simulink model "ControlSystems16"  (R2020b)
settings: Solver=VariableStepAuto  StartTime=0.0  StopTime=155  FixedStep=0.001  MinStep=1e-5
undefined symbols (not defined in the file): DiscIntNeverNeededParam, magnitude
libraries: pid_lib x3, simulink x3
settings Model: Creator=markb  LastModifiedBy=orangejuzi
settings SolverCC: ShapePreserveControl=EnableAll  AlgebraicLoopSolver=LineSearch  MinimalZcImpactIntegration=on
settings DebuggingCC: ReadBeforeWriteMsg=DisableAll  WriteAfterWriteMsg=DisableAll  WriteAfterReadMsg=DisableAll  MaxConsecutiveZCsMsg=warning  MultiTaskDSMMsg=none  ModelReferenceExtraNoncontSigs=warning
settings ModelReferenceCC: UpdateModelReferenceTargets=IfOutOfDate
settings SFSimCC: SFSimEcho=off

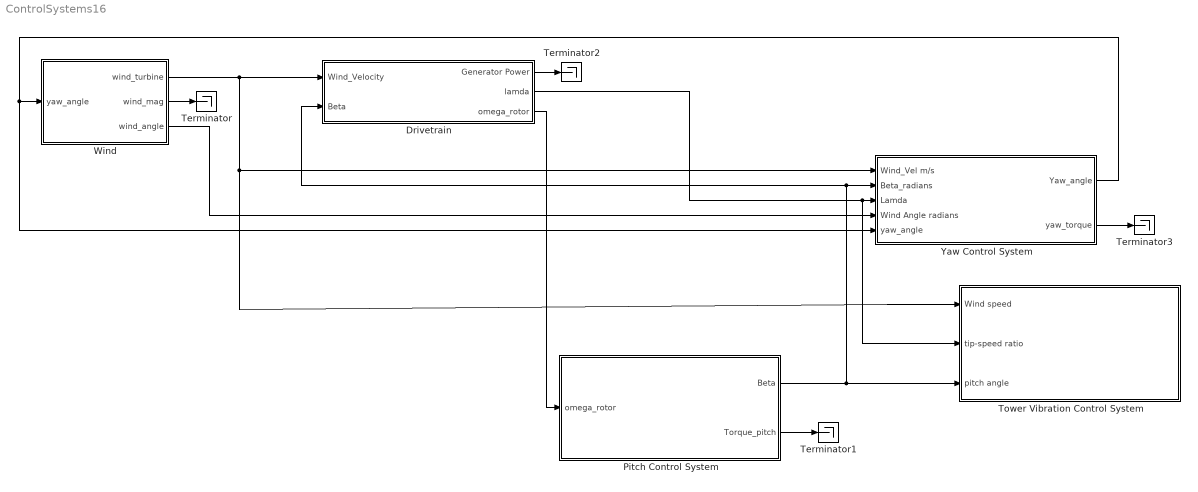
== system ControlSystems16 ==
  Drivetrain : Subsystem
  Pitch Control System : Subsystem
  Terminator{,1..3} (4 alike) : Terminator
  Tower Vibration Control System : Subsystem
  Wind : Subsystem
  Yaw Control System : Subsystem
  wires:
  Yaw Control System/1(Yaw_angle) -> Yaw Control System/5(yaw_angle), Wind/1(yaw_angle)
  Wind/2(wind_mag) -> Terminator/1
  Pitch Control System/1(Beta) -> Drivetrain/2(Beta), Yaw Control System/2(Beta_radians), Tower Vibration Control System/3("pitch angle ")
  Drivetrain/1(Generator Power) -> Terminator2/1
  Wind/3(wind_angle) -> Yaw Control System/4(Wind Angle radians)
  Wind/1(wind_turbine) -> Drivetrain/1(Wind_Velocity), Tower Vibration Control System/1(Wind speed), Yaw Control System/1(Wind_Vel m/s)
  Pitch Control System/2(Torque_pitch) -> Terminator1/1
  Yaw Control System/2(yaw_torque) -> Terminator3/1
  Drivetrain/2(lamda) -> Tower Vibration Control System/2(tip-speed ratio), Yaw Control System/3(Lamda)
  Drivetrain/3(omega_rotor) -> Pitch Control System/1(omega_rotor)

== system ControlSystems16/Drivetrain ==
  Wind_Velocity : Inport
  Beta : Inport  Port=2
  Aerodynamic Block : Subsystem
  Electricl Block : Subsystem
  Mechanical Bock : Subsystem
  Generator Power : Outport
  lamda : Outport  Port=2
  omega_rotor : Outport  Port=3
  wires:
  Mechanical Bock/2(omega_Gen) -> Electricl Block/1(HSS_Speed)
  Electricl Block/2(Generator Torque) -> Mechanical Bock/2(Gen_Torque)
  Mechanical Bock/1(omega_rotor) -> omega_rotor/1, Aerodynamic Block/1(Rotor_Angular_Velocity)
  Wind_Velocity/1 -> Aerodynamic Block/2(Wind_Velocity)
  Beta/1 -> Aerodynamic Block/3(Beta)
  Aerodynamic Block/2(lamda) -> lamda/1
  Aerodynamic Block/1(Rotor_Torque) -> Mechanical Bock/1(Rotor_Torque)
  Electricl Block/1(Generator Power) -> Generator Power/1

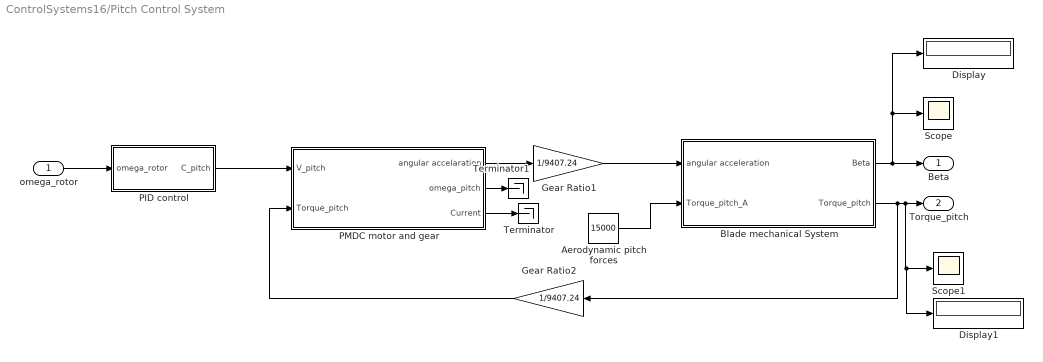
== system ControlSystems16/Pitch Control System ==
  omega_rotor : Inport
  Aerodynamic pitch forces : Constant  Value=15000
  Blade mechanical System : Subsystem
  Display : Display
  Display1 : Display
  Gear Ratio1 : Gain  Gain=1/9407.24
  Gear Ratio2 : Gain  Gain=1/9407.24
  PID control : Subsystem
  PMDC motor and gear : Subsystem
  Scope : Scope
  Scope1 : Scope
  Terminator : Terminator
  Terminator1 : Terminator
  Beta : Outport
  Torque_pitch : Outport  Port=2
  wires:
  omega_rotor/1 -> PID control/1(omega_rotor)
  Aerodynamic pitch forces/1 -> Blade mechanical System/2(Torque_pitch_A)
  Blade mechanical System/2(Torque_pitch) -> Display1/1, Scope1/1, Torque_pitch/1, Gear Ratio2/1
  PID control/1(C_pitch) -> PMDC motor and gear/1(V_pitch)
  Blade mechanical System/1(Beta) -> Display/1, Scope/1, Beta/1
  Gear Ratio1/1 -> Blade mechanical System/1(angular acceleration)
  Gear Ratio2/1 -> PMDC motor and gear/2(Torque_pitch)
  PMDC motor and gear/1(angular accelaration) -> Gear Ratio1/1
  PMDC motor and gear/3(Current) -> Terminator/1
  PMDC motor and gear/2(omega_pitch) -> Terminator1/1

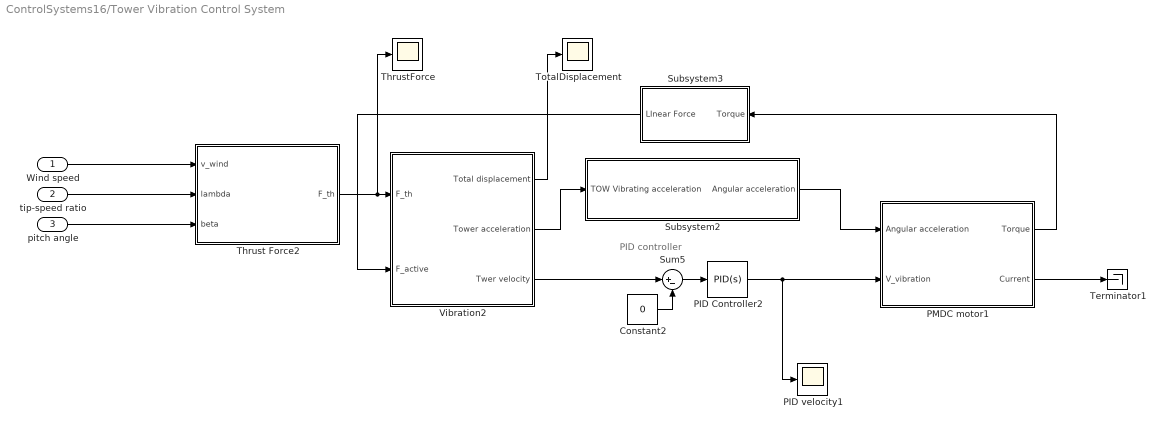
== system ControlSystems16/Tower Vibration Control System ==
  note: PID controller
  Wind speed : Inport
  tip-speed ratio : Inport  Port=2
  "pitch angle " : Inport  Port=3
  Constant2 : Constant  Value=0
  PID Controller2 : pid_lib/PID Controller  Controller=PID  Form=Parallel  TimeDomain=Continuous-time  UseExternalTs=off  SampleTime=-1  IntegratorMethod=Forward Euler  FilterMethod=Forward Euler  ControllerParametersSource=internal  P=-2000  I=-1  D=-1  UseFilter=on  N=597.035100888721  TunerSelectOption=Transfer Function Based (PID Tuner App)  InitialConditionSource=internal  InitialConditionForIntegrator=0  InitialConditionForFilter=0  DifferentiatorICPrevScaledInput=0  ExternalReset=none  TrackingMode=off  Kt=1  LimitOutput=off  SatLimitsSource=internal  UpperSaturationLimit=inf  LowerSaturationLimit=-inf  LinearizeAsGain=on  AntiWindupMode=none  Kb=1  POutMin=[]  POutMax=[]  IOutMin=[]  IOutMax=[]  DOutMin=[]  DOutMax=[]  NOutMin=[]  NOutMax=[]  SumOutMin=[]  SumOutMax=[]  SaturationOutMin=[]  SaturationOutMax=[]  PParamMin=[]  PParamMax=[]  IParamMin=[]  IParamMax=[]  DParamMin=[]  DParamMax=[]  NParamMin=[]  NParamMax=[]  KbParamMin=[]  KbParamMax=[]  KtParamMin=[]  KtParamMax=[]  KbOutMin=[]  KbOutMax=[]  KtOutMin=[]  KtOutMax=[]  IntegratorOutMin=[]  IntegratorOutMax=[]  FilterOutMin=[]  FilterOutMax=[]  SumI1OutMin=[]  SumI1OutMax=[]  SumI2OutMin=[]  SumI2OutMax=[]  SumI3OutMin=[]  SumI3OutMax=[]  SumI4OutMin=[]  SumI4OutMax=[]  SumDOutMin=[]  SumDOutMax=[]  DifferentiatorOutMin=[]  DifferentiatorOutMax=[]  FilterDiffOutCoefMin=[]  FilterDiffOutCoefMax=[]  ReciprocalOutMin=[]  ReciprocalOutMax=[]  SumDenOutMin=[]  SumDenOutMax=[]  SumNumOutMin=[]  SumNumOutMax=[]  DivideOutMin=[]  DivideOutMax=[]  UdiffTsProdOutMin=[]  UdiffTsProdOutMax=[]  NTsProdOutMin=[]  NTsProdOutMax=[]  UintegralTsProdOutMin=[]  UintegralTsProdOutMax=[]  UngainTsProdOutMin=[]  UngainTsProdOutMax=[]  IntegratorContinuousStateAttributes=''  IntegratorStateMustResolveToSignalObject=off  IntegratorRTWStateStorageClass=Auto  FilterContinuousStateAttributes=''  FilterStateMustResolveToSignalObject=off  FilterRTWStateStorageClass=Auto  ParallelPVariant=InternalParameters  IdealPVariant=Disabled  IVariant=InternalParameters  DVariant=InternalParameters  IntegratorVariant=Continuous  SatVariant=Disabled  AWVariant=Passthrough  PCopyVariant=Disabled  TRVariant=Disabled  FdbkBlocksVariant=Forward  IdealPFdbkVariant=Disabled  SatFdbkVariant=Disabled  DerivativeFilterVariant=ContFilter  NVariant=InternalParameters  NCopyVariant=Disabled  FilterICVariant=InternalICsFilter  IntegratorICVariant=InternalICs  ExternalResetVariant=Disabled  TRSumVariant=Passthrough  SumFdbkVariant=Disabled  SumVariant=Sum_PID  TsampFilterVariant=InternalTs  TsampNgainVariant=Passthrough  TsampIntegralVariant=Passthrough  ExternalSaturationOutDataTypeStr=Inherit: Same as second input
  PID velocity1 : Scope
  PMDC motor1 : Subsystem
  Subsystem2 : Subsystem
  Subsystem3 : Subsystem
  Sum5 : Sum  Inputs=|+-
  Terminator1 : Terminator
  Thrust Force2 : Subsystem
  ThrustForce : Scope
  TotalDisplacement : Scope
  Vibration2 : Subsystem
  wires:
  Wind speed/1 -> Thrust Force2/1(v_wind)
  "pitch angle "/1 -> Thrust Force2/3(beta)
  tip-speed ratio/1 -> Thrust Force2/2(lambda)
  PMDC motor1/2(Current) -> Terminator1/1
  Subsystem2/1(Angular acceleration) -> PMDC motor1/1(Angular acceleration)
  Sum5/1 -> PID Controller2/1
  Constant2/1 -> Sum5/2
  Vibration2/3(Twer velocity) -> Sum5/1
  PID Controller2/1 -> PID velocity1/1, PMDC motor1/2(V_vibration)
  PMDC motor1/1(Torque) -> Subsystem3/1(Torque)
  Vibration2/2(Tower acceleration) -> Subsystem2/1(TOW Vibrating acceleration)
  Thrust Force2/1(F_th) -> ThrustForce/1, Vibration2/1(F_th)
  Vibration2/1(Total displacement) -> TotalDisplacement/1
  Subsystem3/1(LInear Force) -> Vibration2/2(F_active)

== system ControlSystems16/Wind ==
  yaw_angle : Inport
  Add : Sum  Inputs=-+
  Product : Product
  Ramp_for_wind_test : simulink/Sources/Ramp  slope=0.1  start=0  InitialOutput=10
  Terminator : Terminator
  Trigonometric Function : Trigonometry  Operator=cos
  Wind_mag : simulink/Sources/Repeating Sequence Interpolated  OutValues=[6 10 15 10 10 15 18 20 22 26 20 22 18 15 13 13 12 10 9 11 17 17 19 19 25 25 26 19 13 10 7 ].'  TimeValues=[0 5 15 20 25 30 35 40 45 50 55 60 65 70 75 80 85 90 95 100 105 110 115 120 125 130 135 140 145 150 155 ].'  LookUpMeth=Interpolation-Use End Values  tsamp=0.01  OutMin=[]  OutMax=[]  OutDataTypeStr=double  OutputDataTypeScalingMode=double  OutDataType=fixdt(0,8)  OutScaling=2^-10
  deg_to_rad : Gain  Gain=pi/180
  omega_w_deg : simulink/Sources/Repeating Sequence Interpolated  OutValues=[ 0 0 0 6 10 12 12 4 8 12 16 16 24 28 24 16 12 4 2 0 0 -2 -4 -4 -10 -14 -18 -20 -12 -8 -4 ].'  TimeValues=[0 5 15 20 25 30 35 40 45 50 55 60 65 70 75 80 85 90 95 100 105 110 115 120 125 130 135 140 145 150 155 ].'  LookUpMeth=Interpolation-Use End Values  tsamp=0.01  OutMin=[]  OutMax=[]  OutDataTypeStr=double  OutputDataTypeScalingMode=double  OutDataType=fixdt(0,8)  OutScaling=2^-10
  wind_turbine : Outport
  wind_mag : Outport  Port=2
  wind_angle : Outport  Port=3
  wires:
  Add/1 -> Trigonometric Function/1
  Trigonometric Function/1 -> Product/1
  deg_to_rad/1 -> wind_angle/1, Add/2
  yaw_angle/1 -> Add/1
  omega_w_deg/1 -> deg_to_rad/1
  Wind_mag/1 -> wind_mag/1, Product/2
  Product/1 -> wind_turbine/1
  Ramp_for_wind_test/1 -> Terminator/1

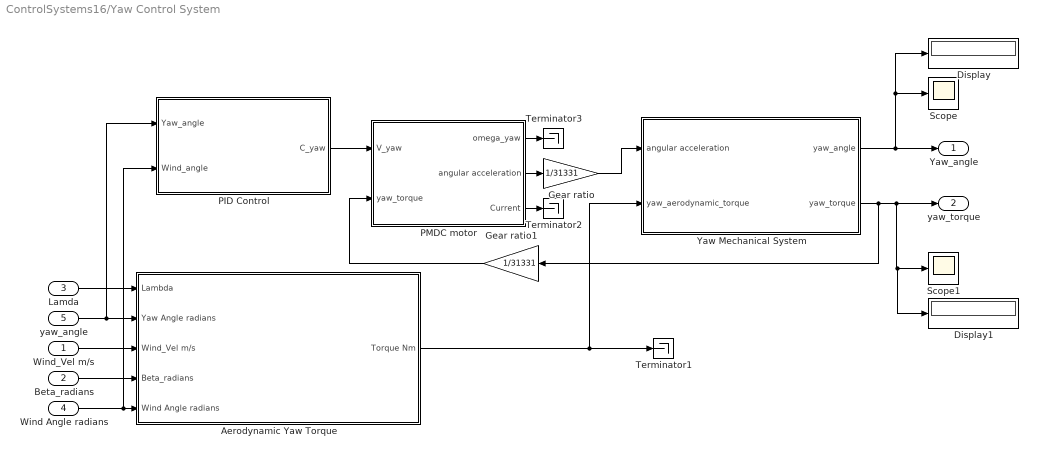
== system ControlSystems16/Yaw Control System ==
  Wind_Vel m/s : Inport
  Beta_radians : Inport  Port=2
  Lamda : Inport  Port=3
  Wind Angle radians : Inport  Port=4
  yaw_angle : Inport  Port=5
  Aerodynamic Yaw Torque : Subsystem
  Display : Display
  Display1 : Display
  Gear ratio : Gain  Gain=1/31331
  Gear ratio1 : Gain  Gain=1/31331
  PID Control : Subsystem
  PMDC motor : Subsystem
  Scope : Scope
  Scope1 : Scope
  Terminator1 : Terminator
  Terminator2 : Terminator
  Terminator3 : Terminator
  Yaw Mechanical System : Subsystem
  Yaw_angle : Outport
  yaw_torque : Outport  Port=2
  wires:
  Wind_Vel m/s/1 -> Aerodynamic Yaw Torque/3(Wind_Vel m/s)
  Wind Angle radians/1 -> PID Control/2(Wind_angle), Aerodynamic Yaw Torque/5(Wind Angle radians)
  Beta_radians/1 -> Aerodynamic Yaw Torque/4(Beta_radians)
  Lamda/1 -> Aerodynamic Yaw Torque/1(Lambda)
  Aerodynamic Yaw Torque/1(Torque Nm) -> Terminator1/1, Yaw Mechanical System/2(yaw_aerodynamic_torque)
  yaw_angle/1 -> Aerodynamic Yaw Torque/2(Yaw Angle radians), PID Control/1(Yaw_angle)
  PID Control/1(C_yaw) -> PMDC motor/1(V_yaw)
  Yaw Mechanical System/2(yaw_torque) -> Display1/1, Scope1/1, yaw_torque/1, Gear ratio1/1
  Yaw Mechanical System/1(yaw_angle) -> Display/1, Scope/1, Yaw_angle/1
  PMDC motor/3(Current) -> Terminator2/1
  PMDC motor/2(angular acceleration) -> Gear ratio/1
  Gear ratio/1 -> Yaw Mechanical System/1(angular acceleration)
  Gear ratio1/1 -> PMDC motor/2(yaw_torque)
  PMDC motor/1(omega_yaw) -> Terminator3/1

== system ControlSystems16/Drivetrain/Aerodynamic Block ==
  Rotor_Angular_Velocity : Inport
  Wind_Velocity : Inport  Port=2
  Beta : Inport  Port=3
  Power Coefficient : Subsystem
  Rotor Torque : Subsystem
  Tip speed Ratio : Subsystem
  Rotor_Torque : Outport
  lamda : Outport  Port=2
  wires:
  Beta/1 -> Power Coefficient/2(Beta)
  Tip speed Ratio/1(Tip_Speed_Ratio) -> lamda/1, Power Coefficient/1(Lamda)
  Power Coefficient/1(C_p) -> Rotor Torque/1(Power_Coefficient)
  Rotor_Angular_Velocity/1 -> Rotor Torque/3(Rotor_Angular_Velocity), Tip speed Ratio/1(Rotor_Angular_Velocity)
  Rotor Torque/1(Rotor_Torque) -> Rotor_Torque/1
  Wind_Velocity/1 -> Rotor Torque/2(Wind_Speed), Tip speed Ratio/2(Wind_Velocity)

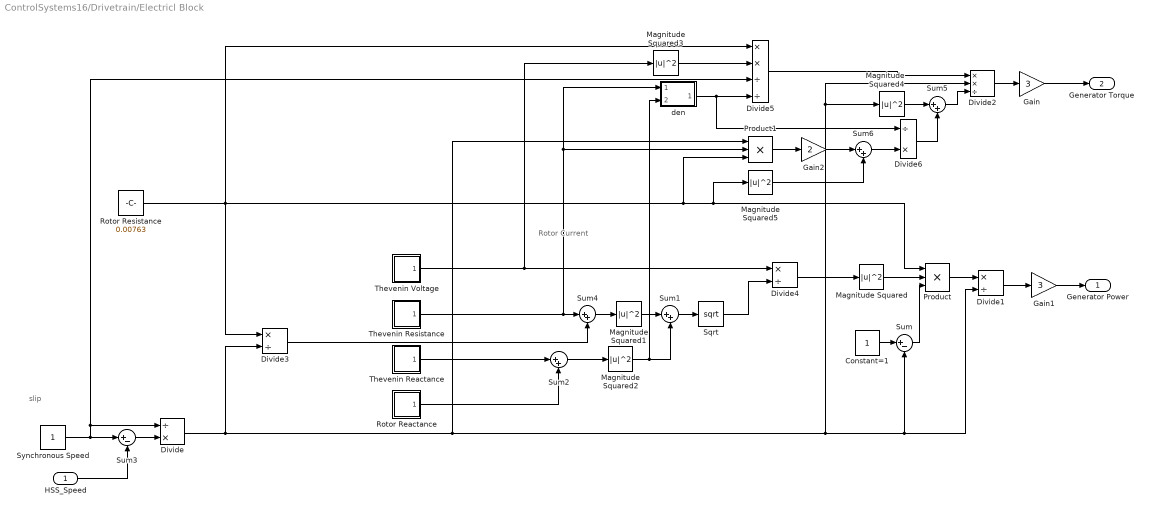
== system ControlSystems16/Drivetrain/Electricl Block ==
  note: slip
  note: Rotor Current
  HSS_Speed : Inport
  Constant=1 : Constant
  Divide : Product  Inputs=/*
  Divide1 : Product  Inputs=*/
  Divide2 : Product  Inputs=**/
  Divide3 : Product  Inputs=*/
  Divide4 : Product  Inputs=*/
  Divide5 : Product  Inputs=**//
  Divide6 : Product  Inputs=/*
  Gain : Gain  Gain=3
  Gain1 : Gain  Gain=3
  Gain2 : Gain  Gain=2
  Magnitude Squared{,1..5} (6 alike) : Math  Operator=magnitude^2  SaturateOnIntegerOverflow=on
  Product : Product  Inputs=3
  Product1 : Product  Inputs=3
  Rotor Reactance : Subsystem
  Rotor Resistance : Constant  Value=0.00763
  Sqrt : Sqrt  SaturateOnIntegerOverflow=on
  Sum : Sum  Inputs=|+-
  Sum{1..2,4..6} (5 alike) : Sum  Inputs=|++
  Sum3 : Sum  Inputs=|+-
  Synchronous Speed : Constant
  Thevenin Reactance : Subsystem
  Thevenin Resistance : Subsystem
  Thevenin Voltage : Subsystem
  den : Subsystem
  Generator Power : Outport
  Generator Torque : Outport  Port=2
  wires:
  Product/1 -> Divide1/1
  Divide1/1 -> Gain1/1
  Gain1/1 -> Generator Power/1
  Sum/1 -> Product/3
  Divide/1 -> Product1/1, Divide1/2, Sum/2, Magnitude Squared4/1, Divide2/2, Divide3/2
  Constant=1/1 -> Sum/1
  Rotor Resistance/1 -> Product1/3, Product/1, Magnitude Squared5/1, Divide3/1, Divide5/1
  Divide4/1 -> Magnitude Squared/1
  Magnitude Squared/1 -> Product/2
  Gain/1 -> Generator Torque/1
  Divide2/1 -> Gain/1
  Thevenin Voltage/1(Out1) -> Magnitude Squared3/1, Divide4/1
  Divide3/1 -> Sum4/2
  Magnitude Squared2/1 -> Sum1/2, den/2(In2)
  Magnitude Squared1/1 -> Sum1/1
  Sqrt/1 -> Divide4/2
  Sum2/1 -> Magnitude Squared2/1
  Thevenin Reactance/1(Out1) -> Sum2/1
  Sum1/1 -> Sqrt/1
  Magnitude Squared3/1 -> Divide5/2
  Synchronous Speed/1 -> Divide5/3, Divide/1, Sum3/1
  HSS_Speed/1 -> Sum3/2
  Sum3/1 -> Divide/2
  Divide5/1 -> Divide2/1
  den/1(Out1) -> Divide6/1, Divide5/4
  Sum4/1 -> Magnitude Squared1/1
  Sum5/1 -> Divide2/3
  Magnitude Squared4/1 -> Sum5/1
  Divide6/1 -> Sum5/2
  Sum6/1 -> Divide6/2
  Gain2/1 -> Sum6/1
  Product1/1 -> Gain2/1
  Magnitude Squared5/1 -> Sum6/2
  Rotor Reactance/1(Out1) -> Sum2/2
  Thevenin Resistance/1(Out1) -> Sum4/1, Product1/2, den/1(In1)

== system ControlSystems16/Drivetrain/Mechanical Bock ==
  Rotor_Torque : Inport
  Gen_Torque : Inport  Port=2
  Discrete-Time Integrator : DiscreteIntegrator  InitialCondition=1.9  SampleTime=-1  ICPrevOutput=DiscIntNeverNeededParam  ICPrevScaledInput=DiscIntNeverNeededParam
  Gain1 : Gain  Gain=1/(2953248-56.442*80^2)
  Gain2 : Gain  Gain=(2953248-56.442*80^2)/(10-1.6*80^2)
  Gear ratio : Gain  Gain=80
  Gear ratio1 : Gain  Gain=80
  Scope : Scope
  Sum : Sum  Inputs=|+--
  omega_rotor : Outport
  omega_Gen : Outport  Port=2
  wires:
  Rotor_Torque/1 -> Sum/1
  Gen_Torque/1 -> Gear ratio/1
  Gear ratio/1 -> Sum/2
  Gain2/1 -> Sum/3
  Gear ratio1/1 -> omega_Gen/1
  Discrete-Time Integrator/1 -> omega_rotor/1, Scope/1, Gear ratio1/1, Gain2/1
  Sum/1 -> Gain1/1
  Gain1/1 -> Discrete-Time Integrator/1

== system ControlSystems16/Pitch Control System/Blade mechanical System ==
  angular acceleration : Inport
  Torque_pitch_A : Inport  Port=2
  Add : Sum  Inputs=++-
  D_pitch : Gain  Gain=100
  Integrator : Integrator
  Integrator1 : Integrator
  Integrator2 : Integrator
  J_pitch : Gain  Gain=22800
  Beta : Outport
  Torque_pitch : Outport  Port=2
  wires:
  Integrator/1 -> Beta/1
  Add/1 -> Torque_pitch/1
  Torque_pitch_A/1 -> Add/3
  D_pitch/1 -> Add/2
  J_pitch/1 -> Add/1
  angular acceleration/1 -> J_pitch/1, Integrator1/1, Integrator2/1
  Integrator1/1 -> D_pitch/1
  Integrator2/1 -> Integrator/1

== system ControlSystems16/Pitch Control System/PID control ==
  omega_rotor : Inport
  Constant : Constant
  PID Controller : pid_lib/PID Controller  Controller=PID  Form=Parallel  TimeDomain=Continuous-time  UseExternalTs=off  SampleTime=-1  IntegratorMethod=Forward Euler  FilterMethod=Forward Euler  ControllerParametersSource=internal  P=1  I=1  D=0  UseFilter=on  N=100  TunerSelectOption=Transfer Function Based (PID Tuner App)  InitialConditionSource=internal  InitialConditionForIntegrator=0  InitialConditionForFilter=0  DifferentiatorICPrevScaledInput=0  ExternalReset=none  TrackingMode=off  Kt=1  LimitOutput=off  SatLimitsSource=internal  UpperSaturationLimit=inf  LowerSaturationLimit=-inf  LinearizeAsGain=on  AntiWindupMode=none  Kb=1  POutMin=[]  POutMax=[]  IOutMin=[]  IOutMax=[]  DOutMin=[]  DOutMax=[]  NOutMin=[]  NOutMax=[]  SumOutMin=[]  SumOutMax=[]  SaturationOutMin=[]  SaturationOutMax=[]  PParamMin=[]  PParamMax=[]  IParamMin=[]  IParamMax=[]  DParamMin=[]  DParamMax=[]  NParamMin=[]  NParamMax=[]  KbParamMin=[]  KbParamMax=[]  KtParamMin=[]  KtParamMax=[]  KbOutMin=[]  KbOutMax=[]  KtOutMin=[]  KtOutMax=[]  IntegratorOutMin=[]  IntegratorOutMax=[]  FilterOutMin=[]  FilterOutMax=[]  SumI1OutMin=[]  SumI1OutMax=[]  SumI2OutMin=[]  SumI2OutMax=[]  SumI3OutMin=[]  SumI3OutMax=[]  SumI4OutMin=[]  SumI4OutMax=[]  SumDOutMin=[]  SumDOutMax=[]  DifferentiatorOutMin=[]  DifferentiatorOutMax=[]  FilterDiffOutCoefMin=[]  FilterDiffOutCoefMax=[]  ReciprocalOutMin=[]  ReciprocalOutMax=[]  SumDenOutMin=[]  SumDenOutMax=[]  SumNumOutMin=[]  SumNumOutMax=[]  DivideOutMin=[]  DivideOutMax=[]  UdiffTsProdOutMin=[]  UdiffTsProdOutMax=[]  NTsProdOutMin=[]  NTsProdOutMax=[]  UintegralTsProdOutMin=[]  UintegralTsProdOutMax=[]  UngainTsProdOutMin=[]  UngainTsProdOutMax=[]  IntegratorContinuousStateAttributes=''  IntegratorStateMustResolveToSignalObject=off  IntegratorRTWStateStorageClass=Auto  FilterContinuousStateAttributes=''  FilterStateMustResolveToSignalObject=off  FilterRTWStateStorageClass=Auto  ParallelPVariant=InternalParameters  IdealPVariant=Disabled  IVariant=InternalParameters  DVariant=InternalParameters  IntegratorVariant=Continuous  SatVariant=Disabled  AWVariant=Passthrough  PCopyVariant=Disabled  TRVariant=Disabled  FdbkBlocksVariant=Forward  IdealPFdbkVariant=Disabled  SatFdbkVariant=Disabled  DerivativeFilterVariant=ContFilter  NVariant=InternalParameters  NCopyVariant=Disabled  FilterICVariant=InternalICsFilter  IntegratorICVariant=InternalICs  ExternalResetVariant=Disabled  TRSumVariant=Passthrough  SumFdbkVariant=Disabled  SumVariant=Sum_PID  TsampFilterVariant=InternalTs  TsampNgainVariant=Passthrough  TsampIntegralVariant=Passthrough  ExternalSaturationOutDataTypeStr=Inherit: Same as second input
  Sum : Sum  Inputs=|+-
  C_pitch : Outport
  wires:
  omega_rotor/1 -> Sum/1
  PID Controller/1 -> C_pitch/1
  Sum/1 -> PID Controller/1
  Constant/1 -> Sum/2

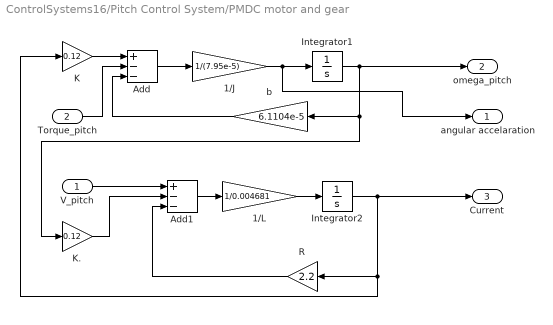
== system ControlSystems16/Pitch Control System/PMDC motor and gear ==
  V_pitch : Inport
  Torque_pitch : Inport  Port=2
  1/J : Gain  Gain=1/(7.95e-5)
  1/L : Gain  Gain=1/0.004681
  Add : Sum  Inputs=+--
  Add1 : Sum  Inputs=+--
  Integrator1 : Integrator
  Integrator2 : Integrator
  K : Gain  Gain=0.12
  K. : Gain  Gain=0.12
  R : Gain  Gain=2.2
  b : Gain  Gain=6.1104e-5
  angular accelaration : Outport
  omega_pitch : Outport  Port=2
  Current : Outport  Port=3
  wires:
  K/1 -> Add/1
  K./1 -> Add1/2
  Add1/1 -> 1/L/1
  Torque_pitch/1 -> Add/2
  Integrator1/1 -> omega_pitch/1, K./1, b/1
  1/L/1 -> Integrator2/1
  1/J/1 -> angular accelaration/1, Integrator1/1
  R/1 -> Add1/3
  Add/1 -> 1/J/1
  Integrator2/1 -> Current/1, R/1, K/1
  V_pitch/1 -> Add1/1
  b/1 -> Add/3

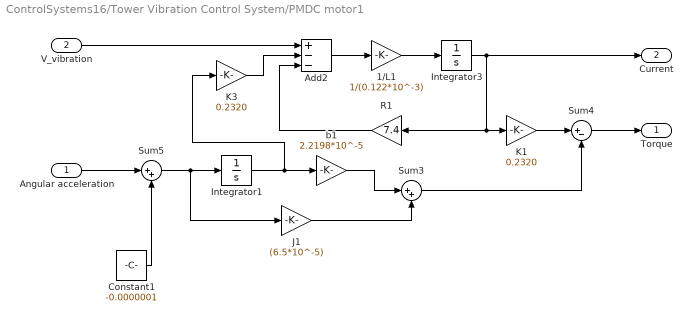
== system ControlSystems16/Tower Vibration Control System/PMDC motor1 ==
  Angular acceleration : Inport
  V_vibration : Inport  Port=2
  1/L1 : Gain  Gain=1/(0.122*10^-3)
  Add2 : Sum  Inputs=+--
  Constant1 : Constant  Value=-0.0000001
  Integrator1 : Integrator
  Integrator3 : Integrator
  J1 : Gain  Gain=(6.5*10^-5)
  K1 : Gain  Gain=0.2320
  K3 : Gain  Gain=0.2320
  R1 : Gain  Gain=7.4
  Sum3 : Sum  Inputs=|++
  Sum4 : Sum  Inputs=|+-
  Sum5 : Sum  Inputs=|++
  b1 : Gain  Gain=2.2198*10^-5
  Torque : Outport
  Current : Outport  Port=2
  wires:
  K3/1 -> Add2/2
  Sum4/1 -> Torque/1
  Add2/1 -> 1/L1/1
  K1/1 -> Sum4/1
  V_vibration/1 -> Add2/1
  Integrator3/1 -> Current/1, R1/1, K1/1
  Constant1/1 -> Sum5/2
  Sum5/1 -> J1/1, Integrator1/1
  Integrator1/1 -> K3/1, b1/1
  1/L1/1 -> Integrator3/1
  b1/1 -> Sum3/1
  Sum3/1 -> Sum4/2
  R1/1 -> Add2/3
  J1/1 -> Sum3/2
  Angular acceleration/1 -> Sum5/1

== system ControlSystems16/Tower Vibration Control System/Subsystem2 ==
  TOW Vibrating acceleration : Inport
  GearRatio : Gain  Gain=1/300
  Angular acceleration : Outport
  wires:
  TOW Vibrating acceleration/1 -> GearRatio/1
  GearRatio/1 -> Angular acceleration/1

== system ControlSystems16/Tower Vibration Control System/Subsystem3 ==
  Torque : Inport
  Raduis : Gain  Gain=4000*0.5
  LInear Force : Outport
  wires:
  Torque/1 -> Raduis/1
  Raduis/1 -> LInear Force/1

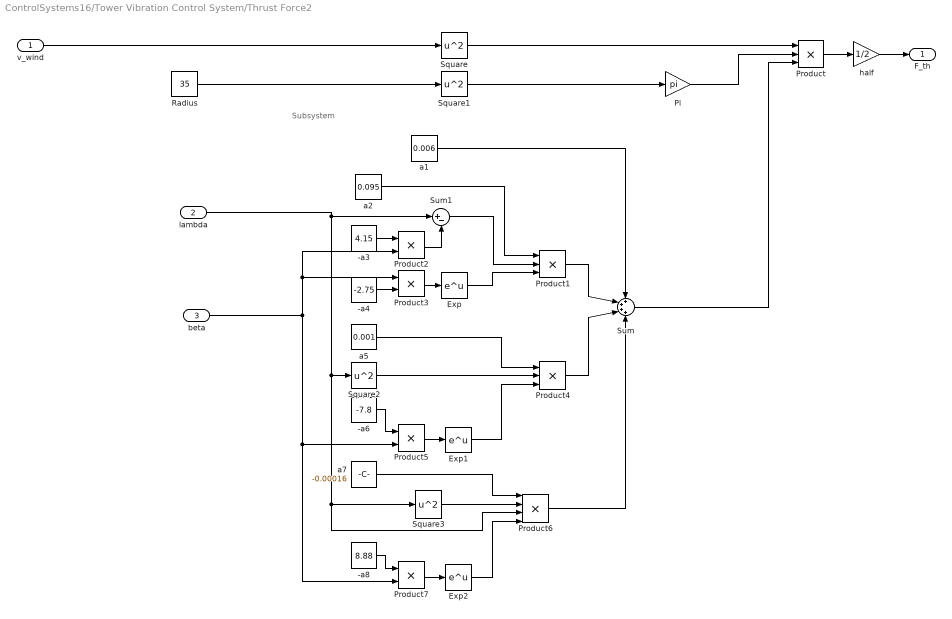
== system ControlSystems16/Tower Vibration Control System/Thrust Force2 ==
  note: Subsystem
  v_wind : Inport
  lambda : Inport  Port=2
  beta : Inport  Port=3
  -a3 : Constant  Value=4.15
  -a4 : Constant  Value=-2.75
  -a6 : Constant  Value=-7.8
  -a8 : Constant  Value=8.88
  Exp : Math  SaturateOnIntegerOverflow=on
  Exp1 : Math  SaturateOnIntegerOverflow=on
  Exp2 : Math  SaturateOnIntegerOverflow=on
  Pi : Gain  Gain=pi
  Product : Product  Inputs=3
  Product1 : Product  Inputs=3
  Product{2..3,5,7} (4 alike) : Product
  Product4 : Product  Inputs=3
  Product6 : Product  Inputs=4
  Radius : Constant  Value=35
  Square{,1..3} (4 alike) : Math  Operator=square  SaturateOnIntegerOverflow=on
  Sum : Sum  Inputs=4
  Sum1 : Sum  Inputs=|+-
  a1 : Constant  Value=0.006
  a2 : Constant  Value=0.095
  a5 : Constant  Value=0.001
  a7 : Constant  Value=-0.00016
  half : Gain  Gain=1/2
  F_th : Outport
  wires:
  v_wind/1 -> Square/1
  half/1 -> F_th/1
  Product/1 -> half/1
  Square/1 -> Product/1
  Radius/1 -> Square1/1
  Square1/1 -> Pi/1
  Pi/1 -> Product/2
  Sum/1 -> Product/3
  Product3/1 -> Exp/1
  Product7/1 -> Exp2/1
  Exp2/1 -> Product6/4
  Exp/1 -> Product1/3
  Product1/1 -> Sum/2
  Product5/1 -> Exp1/1
  lambda/1 -> Square3/1, Product6/3, Square2/1, Sum1/1
  Product2/1 -> Sum1/2
  Product6/1 -> Sum/4
  Exp1/1 -> Product4/3
  Sum1/1 -> Product1/2
  -a6/1 -> Product5/1
  a5/1 -> Product4/1
  Square2/1 -> Product4/2
  a1/1 -> Sum/1
  a2/1 -> Product1/1
  -a8/1 -> Product7/1
  Product4/1 -> Sum/3
  a7/1 -> Product6/1
  -a4/1 -> Product3/2
  -a3/1 -> Product2/1
  beta/1 -> Product5/2, Product7/2, Product3/1, Product2/2
  Square3/1 -> Product6/2

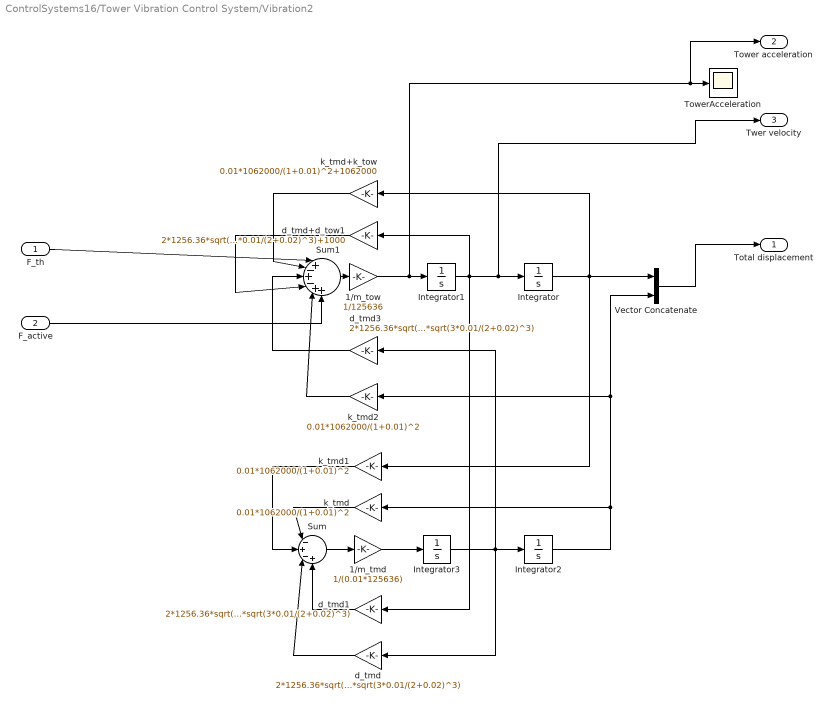
== system ControlSystems16/Tower Vibration Control System/Vibration2 ==
  F_th : Inport
  F_active : Inport  Port=2
  1/m_tmd : Gain  Gain=1/(0.01*125636)
  1/m_tow : Gain  Gain=1/125636
  Integrator : Integrator
  Integrator1 : Integrator  InitialCondition=1.9  UpperSaturationLimit=10  LowerSaturationLimit=-10  AbsoluteTolerance=0.001
  Integrator2 : Integrator
  Integrator3 : Integrator
  Sum : Sum  Inputs=|-+-+
  Sum1 : Sum  Inputs=|+-+-++
  TowerAcceleration : Scope
  Vector Concatenate : Concatenate
  d_tmd : Gain  Gain=2*1256.36*sqrt(1062000/125636)*sqrt(3*0.01/(2+0.02)^3)
  d_tmd+d_tow1 : Gain  Gain=2*1256.36*sqrt(1062000/125636)*sqrt(3*0.01/(2+0.02)^3)+1000
  d_tmd1 : Gain  Gain=2*1256.36*sqrt(1062000/125636)*sqrt(3*0.01/(2+0.02)^3)
  d_tmd3 : Gain  Gain=2*1256.36*sqrt(1062000/125636)*sqrt(3*0.01/(2+0.02)^3)
  k_tmd : Gain  Gain=0.01*1062000/(1+0.01)^2
  k_tmd+k_tow : Gain  Gain=0.01*1062000/(1+0.01)^2+1062000
  k_tmd1 : Gain  Gain=0.01*1062000/(1+0.01)^2
  k_tmd2 : Gain  Gain=0.01*1062000/(1+0.01)^2
  Total displacement : Outport
  Tower acceleration : Outport  Port=2
  Twer velocity : Outport  Port=3
  wires:
  Integrator/1 -> k_tmd+k_tow/1, Vector Concatenate/1, k_tmd1/1
  Integrator3/1 -> d_tmd/1, d_tmd3/1, Integrator2/1
  1/m_tmd/1 -> Integrator3/1
  Sum/1 -> 1/m_tmd/1
  1/m_tow/1 -> Tower acceleration/1, TowerAcceleration/1, Integrator1/1
  Sum1/1 -> 1/m_tow/1
  k_tmd/1 -> Sum/1
  d_tmd/1 -> Sum/3
  d_tmd1/1 -> Sum/4
  k_tmd1/1 -> Sum/2
  k_tmd+k_tow/1 -> Sum1/2
  d_tmd+d_tow1/1 -> Sum1/4
  d_tmd3/1 -> Sum1/3
  Integrator2/1 -> k_tmd/1, k_tmd2/1, Vector Concatenate/2
  k_tmd2/1 -> Sum1/5
  Vector Concatenate/1 -> Total displacement/1
  F_th/1 -> Sum1/1
  F_active/1 -> Sum1/6
  Integrator1/1 -> d_tmd+d_tow1/1, d_tmd1/1, Twer velocity/1, Integrator/1

== system ControlSystems16/Yaw Control System/Aerodynamic Yaw Torque ==
  note: Beta needs to be in radians
  Lambda : Inport
  Yaw Angle radians : Inport  Port=2
  Wind_Vel m/s : Inport  Port=3
  Beta_radians : Inport  Port=4
  Wind Angle radians : Inport  Port=5
  Subtract : Sum  Inputs=+-
  block 1 : Subsystem
  block 2 : Subsystem
  Torque Nm : Outport
  wires:
  block 1/1(C_t) -> block 2/1(Thrust_Coefficient)
  Beta_radians/1 -> block 1/2(beta)
  Wind Angle radians/1 -> Subtract/1
  Yaw Angle radians/1 -> Subtract/2
  Subtract/1 -> block 2/3(Wind Angle difference)
  block 2/1(Yaw_Torque) -> Torque Nm/1
  Lambda/1 -> block 1/1(lambda)
  Wind_Vel m/s/1 -> block 2/2(wind_velocity)

== system ControlSystems16/Yaw Control System/PID Control ==
  Yaw_angle : Inport
  Wind_angle : Inport  Port=2
  Constant : Constant
  PID Controller : pid_lib/PID Controller  Controller=PID  Form=Parallel  TimeDomain=Continuous-time  UseExternalTs=off  SampleTime=-1  IntegratorMethod=Forward Euler  FilterMethod=Forward Euler  ControllerParametersSource=internal  P=3  I=3  D=0  UseFilter=on  N=100  TunerSelectOption=Transfer Function Based (PID Tuner App)  InitialConditionSource=internal  InitialConditionForIntegrator=0  InitialConditionForFilter=0  DifferentiatorICPrevScaledInput=0  ExternalReset=none  TrackingMode=off  Kt=1  LimitOutput=off  SatLimitsSource=internal  UpperSaturationLimit=inf  LowerSaturationLimit=-inf  LinearizeAsGain=on  AntiWindupMode=none  Kb=1  POutMin=[]  POutMax=[]  IOutMin=[]  IOutMax=[]  DOutMin=[]  DOutMax=[]  NOutMin=[]  NOutMax=[]  SumOutMin=[]  SumOutMax=[]  SaturationOutMin=[]  SaturationOutMax=[]  PParamMin=[]  PParamMax=[]  IParamMin=[]  IParamMax=[]  DParamMin=[]  DParamMax=[]  NParamMin=[]  NParamMax=[]  KbParamMin=[]  KbParamMax=[]  KtParamMin=[]  KtParamMax=[]  KbOutMin=[]  KbOutMax=[]  KtOutMin=[]  KtOutMax=[]  IntegratorOutMin=[]  IntegratorOutMax=[]  FilterOutMin=[]  FilterOutMax=[]  SumI1OutMin=[]  SumI1OutMax=[]  SumI2OutMin=[]  SumI2OutMax=[]  SumI3OutMin=[]  SumI3OutMax=[]  SumI4OutMin=[]  SumI4OutMax=[]  SumDOutMin=[]  SumDOutMax=[]  DifferentiatorOutMin=[]  DifferentiatorOutMax=[]  FilterDiffOutCoefMin=[]  FilterDiffOutCoefMax=[]  ReciprocalOutMin=[]  ReciprocalOutMax=[]  SumDenOutMin=[]  SumDenOutMax=[]  SumNumOutMin=[]  SumNumOutMax=[]  DivideOutMin=[]  DivideOutMax=[]  UdiffTsProdOutMin=[]  UdiffTsProdOutMax=[]  NTsProdOutMin=[]  NTsProdOutMax=[]  UintegralTsProdOutMin=[]  UintegralTsProdOutMax=[]  UngainTsProdOutMin=[]  UngainTsProdOutMax=[]  IntegratorContinuousStateAttributes=''  IntegratorStateMustResolveToSignalObject=off  IntegratorRTWStateStorageClass=Auto  FilterContinuousStateAttributes=''  FilterStateMustResolveToSignalObject=off  FilterRTWStateStorageClass=Auto  ParallelPVariant=InternalParameters  IdealPVariant=Disabled  IVariant=InternalParameters  DVariant=InternalParameters  IntegratorVariant=Continuous  SatVariant=Disabled  AWVariant=Passthrough  PCopyVariant=Disabled  TRVariant=Disabled  FdbkBlocksVariant=Forward  IdealPFdbkVariant=Disabled  SatFdbkVariant=Disabled  DerivativeFilterVariant=ContFilter  NVariant=InternalParameters  NCopyVariant=Disabled  FilterICVariant=InternalICsFilter  IntegratorICVariant=InternalICs  ExternalResetVariant=Disabled  TRSumVariant=Passthrough  SumFdbkVariant=Disabled  SumVariant=Sum_PID  TsampFilterVariant=InternalTs  TsampNgainVariant=Passthrough  TsampIntegralVariant=Passthrough  ExternalSaturationOutDataTypeStr=Inherit: Same as second input
  Sum : Sum  Inputs=|-+-
  C_yaw : Outport
  wires:
  Wind_angle/1 -> Sum/2
  Yaw_angle/1 -> Sum/1
  Sum/1 -> PID Controller/1
  Constant/1 -> Sum/3
  PID Controller/1 -> C_yaw/1

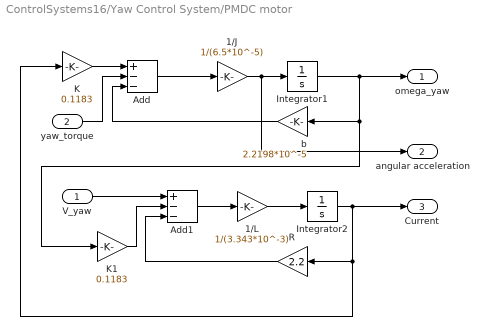
== system ControlSystems16/Yaw Control System/PMDC motor ==
  V_yaw : Inport
  yaw_torque : Inport  Port=2
  1/J : Gain  Gain=1/(6.5*10^-5)
  1/L : Gain  Gain=1/(3.343*10^-3)
  Add : Sum  Inputs=+--
  Add1 : Sum  Inputs=+--
  Integrator1 : Integrator
  Integrator2 : Integrator
  K : Gain  Gain=0.1183
  K1 : Gain  Gain=0.1183
  R : Gain  Gain=2.2
  b : Gain  Gain=2.2198*10^-5
  omega_yaw : Outport
  angular acceleration : Outport  Port=2
  Current : Outport  Port=3
  wires:
  1/J/1 -> angular acceleration/1, Integrator1/1
  Integrator1/1 -> omega_yaw/1, K1/1, b/1
  K1/1 -> Add1/2
  1/L/1 -> Integrator2/1
  yaw_torque/1 -> Add/2
  Add1/1 -> 1/L/1
  K/1 -> Add/1
  Integrator2/1 -> Current/1, R/1, K/1
  b/1 -> Add/3
  Add/1 -> 1/J/1
  V_yaw/1 -> Add1/1
  R/1 -> Add1/3

== system ControlSystems16/Yaw Control System/Yaw Mechanical System ==
  angular acceleration : Inport
  yaw_aerodynamic_torque : Inport  Port=2
  Add : Sum  Inputs=3
  D_yaw : Gain  Gain=200
  Integrator : Integrator
  Integrator1 : Integrator
  Integrator2 : Integrator
  J_yaw : Gain  Gain=45377
  yaw_angle : Outport
  yaw_torque : Outport  Port=2
  wires:
  Integrator/1 -> yaw_angle/1
  Add/1 -> yaw_torque/1
  D_yaw/1 -> Add/2
  yaw_aerodynamic_torque/1 -> Add/3
  J_yaw/1 -> Add/1
  angular acceleration/1 -> Integrator1/1, J_yaw/1, Integrator2/1
  Integrator1/1 -> D_yaw/1
  Integrator2/1 -> Integrator/1

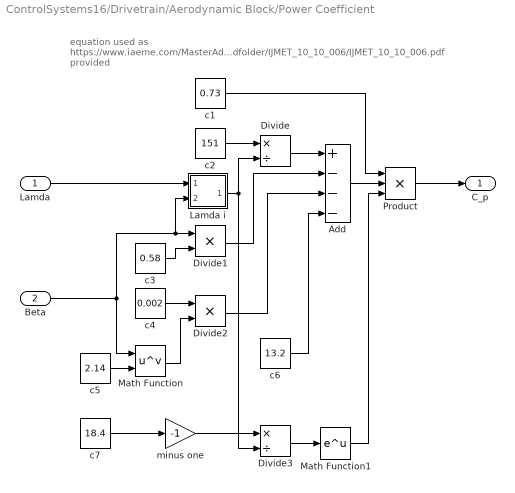
== system ControlSystems16/Drivetrain/Aerodynamic Block/Power Coefficient ==
  note: equation used as
      | https://www.iaeme.com/MasterAdmin/uploadfolder/IJMET_10_10_006/IJMET_10_10_006.pdf provided
  Lamda : Inport
  Beta : Inport  Port=2
  Add : Sum  Inputs=+---
  Divide : Product  Inputs=*/
  Divide1 : Product  Inputs=**
  Divide2 : Product  Inputs=**
  Divide3 : Product  Inputs=*/
  Lamda i : Subsystem
  Math Function : Math  Operator=pow  SaturateOnIntegerOverflow=on
  Math Function1 : Math  SaturateOnIntegerOverflow=on
  Product : Product  Inputs=3
  c1 : Constant  Value=0.73
  c2 : Constant  Value=151
  c3 : Constant  Value=0.58
  c4 : Constant  Value=0.002
  c5 : Constant  Value=2.14
  c6 : Constant  Value=13.2
  c7 : Constant  Value=18.4
  minus one : Gain  Gain=-1
  C_p : Outport
  wires:
  Lamda/1 -> Lamda i/1(In1)
  Beta/1 -> Math Function/1, Divide1/1, Lamda i/2(In2)
  c1/1 -> Product/1
  Product/1 -> C_p/1
  Add/1 -> Product/2
  c2/1 -> Divide/1
  Divide/1 -> Add/1
  Lamda i/1(Out1) -> Divide3/2, Divide/2
  c3/1 -> Divide1/2
  Divide1/1 -> Add/2
  c4/1 -> Divide2/1
  Math Function/1 -> Divide2/2
  c5/1 -> Math Function/2
  Divide2/1 -> Add/3
  c6/1 -> Add/4
  Divide3/1 -> Math Function1/1
  c7/1 -> minus one/1
  minus one/1 -> Divide3/1
  Math Function1/1 -> Product/3

== system ControlSystems16/Drivetrain/Aerodynamic Block/Rotor Torque ==
  note: Power of wind
  Power_Coefficient : Inport
  Wind_Speed : Inport  Port=2
  Rotor_Angular_Velocity : Inport  Port=3
  Divide : Product  Inputs=**/
  Gain : Gain  Gain=0.5*1.225*pi*35^2
  Product : Product
  Square : Math  Operator=square  SaturateOnIntegerOverflow=on
  Rotor_Torque : Outport
  wires:
  Rotor_Angular_Velocity/1 -> Divide/3  "omega_rotor"
  Power_Coefficient/1 -> Divide/1
  Divide/1 -> Rotor_Torque/1
  Wind_Speed/1 -> Square/1, Product/1  "V_wind"
  Gain/1 -> Divide/2
  Product/1 -> Gain/1
  Square/1 -> Product/2

== system ControlSystems16/Drivetrain/Aerodynamic Block/Tip speed Ratio ==
  Rotor_Angular_Velocity : Inport
  Wind_Velocity : Inport  Port=2
  Divide : Product  Inputs=*/
  Radius : Gain  Gain=35
  Tip_Speed_Ratio : Outport
  wires:
  Rotor_Angular_Velocity/1 -> Radius/1  "omega_r"
  Radius/1 -> Divide/1
  Wind_Velocity/1 -> Divide/2  "V_wind"
  Divide/1 -> Tip_Speed_Ratio/1

== system ControlSystems16/Drivetrain/Electricl Block/Rotor Reactance ==
  Gain3 : Gain  Gain=2*pi
  Rotor Inductance : Constant  Value=0.000195
  Out1 : Outport
  wires:
  Gain3/1 -> Out1/1
  Rotor Inductance/1 -> Gain3/1

== system ControlSystems16/Drivetrain/Electricl Block/Thevenin Reactance ==
  Divide7 : Product  Inputs=/**
  Magnitude Squared7 : Math  Operator=magnitude^2  SaturateOnIntegerOverflow=on
  Magnitude Squared8 : Math  Operator=magnitude^2  SaturateOnIntegerOverflow=on
  Mutual Reactance : Subsystem
  Product : Product
  Rotor Resistance1 : Constant  Value=0.00763
  Stator Reactance : Subsystem
  Sum1 : Sum  Inputs=|+-
  Sum7 : Sum  Inputs=|++
  Sum8 : Sum  Inputs=|++
  Out1 : Outport
  wires:
  Sum7/1 -> Divide7/1
  Magnitude Squared7/1 -> Sum1/1, Sum7/1
  Divide7/1 -> Out1/1
  Stator Reactance/1(Out1) -> Product/1, Sum8/1
  Sum8/1 -> Product/2, Magnitude Squared8/1
  Rotor Resistance1/1 -> Magnitude Squared7/1
  Magnitude Squared8/1 -> Sum7/2
  Mutual Reactance/1(Out1) -> Divide7/3, Sum8/2
  Sum1/1 -> Divide7/2
  Product/1 -> Sum1/2

== system ControlSystems16/Drivetrain/Electricl Block/Thevenin Resistance ==
  Divide7 : Product  Inputs=**/
  Magnitude Squared6 : Math  Operator=magnitude^2  SaturateOnIntegerOverflow=on
  Magnitude Squared7 : Math  Operator=magnitude^2  SaturateOnIntegerOverflow=on
  Magnitude Squared8 : Math  Operator=magnitude^2  SaturateOnIntegerOverflow=on
  Mutual Reactance : Subsystem
  Rotor Resistance1 : Constant  Value=0.00763
  Stator Reactance : Subsystem
  Sum7 : Sum  Inputs=|++
  Sum8 : Sum  Inputs=|++
  Out1 : Outport
  wires:
  Sum7/1 -> Divide7/3
  Magnitude Squared7/1 -> Sum7/1
  Divide7/1 -> Out1/1
  Stator Reactance/1(Out1) -> Sum8/2
  Sum8/1 -> Magnitude Squared8/1
  Rotor Resistance1/1 -> Divide7/2, Magnitude Squared7/1
  Magnitude Squared6/1 -> Divide7/1
  Magnitude Squared8/1 -> Sum7/2
  Mutual Reactance/1(Out1) -> Sum8/1, Magnitude Squared6/1

== system ControlSystems16/Drivetrain/Electricl Block/Thevenin Voltage ==
  Divide7 : Product  Inputs=**/
  Divide8 : Product  Inputs=/**
  Magnitude Squared{6..7,9..10} (4 alike) : Math  Operator=magnitude^2  SaturateOnIntegerOverflow=on
  Mutual Reactance : Subsystem
  Rotor Resistance1 : Constant  Value=0.00763
  Sqrt1 : Sqrt  SaturateOnIntegerOverflow=on
  Stator Reactance : Subsystem
  Sum{7..10} (4 alike) : Sum  Inputs=|++
  Out1 : Outport
  wires:
  Sum10/1 -> Divide8/2
  Sum7/1 -> Sqrt1/1
  Sqrt1/1 -> Out1/1
  Mutual Reactance/1(Out1) -> Divide7/2, Sum9/1, Sum10/2, Divide8/3
  Stator Reactance/1(Out1) -> Sum9/2, Sum10/1
  Sum9/1 -> Magnitude Squared10/1
  Magnitude Squared9/1 -> Sum8/1
  Divide8/1 -> Magnitude Squared7/1
  Sum8/1 -> Divide8/1, Divide7/3
  Magnitude Squared10/1 -> Sum8/2
  Magnitude Squared7/1 -> Sum7/2
  Magnitude Squared6/1 -> Sum7/1
  Rotor Resistance1/1 -> Divide7/1, Magnitude Squared9/1
  Divide7/1 -> Magnitude Squared6/1

== system ControlSystems16/Drivetrain/Electricl Block/den ==
  In1 : Inport
  In2 : Inport  Port=2
  Magnitude Squared4 : Math  Operator=magnitude^2  SaturateOnIntegerOverflow=on
  Sum4 : Sum  Inputs=|++
  Out1 : Outport
  wires:
  In2/1 -> Sum4/2
  In1/1 -> Magnitude Squared4/1
  Sum4/1 -> Out1/1
  Magnitude Squared4/1 -> Sum4/1

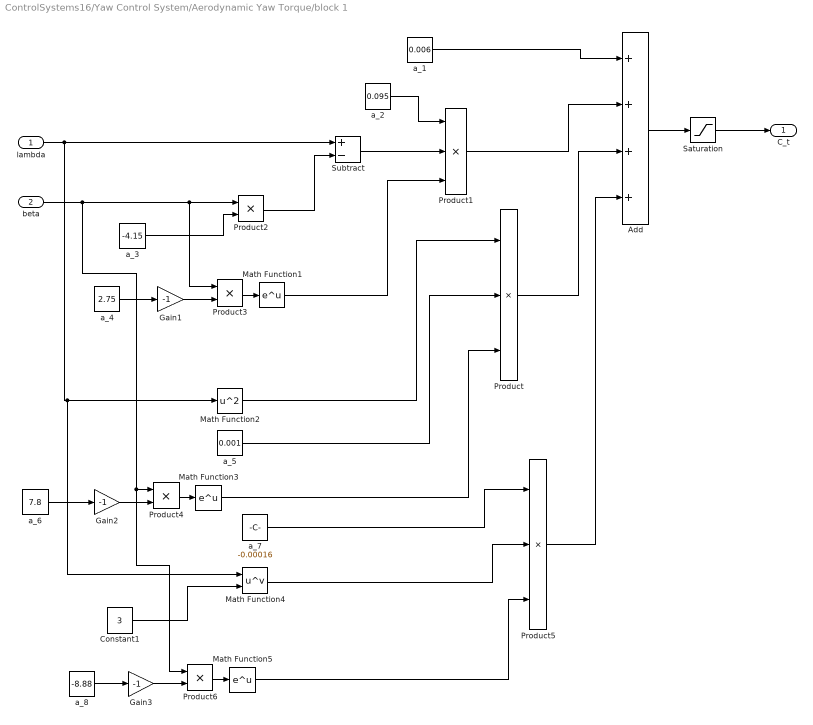
== system ControlSystems16/Yaw Control System/Aerodynamic Yaw Torque/block 1 ==
  lambda : Inport
  beta : Inport  Port=2
  Add : Sum  Inputs=++++
  Constant1 : Constant  Value=3
  Gain1 : Gain  Gain=-1
  Gain2 : Gain  Gain=-1
  Gain3 : Gain  Gain=-1
  Math Function1 : Math  SaturateOnIntegerOverflow=on
  Math Function2 : Math  Operator=square  SaturateOnIntegerOverflow=on
  Math Function3 : Math  SaturateOnIntegerOverflow=on
  Math Function4 : Math  Operator=pow  SaturateOnIntegerOverflow=on
  Math Function5 : Math  SaturateOnIntegerOverflow=on
  Product : Product  Inputs=3
  Product1 : Product  Inputs=3
  Product{2..4,6} (4 alike) : Product
  Product5 : Product  Inputs=3
  Saturation : Saturate  UpperLimit=inf  LowerLimit=0
  Subtract : Sum  Inputs=+-
  a_1 : Constant  Value=0.006
  a_2 : Constant  Value=0.095
  a_3 : Constant  Value=-4.15
  a_4 : Constant  Value=2.75
  a_5 : Constant  Value=0.001
  a_6 : Constant  Value=7.8
  a_7 : Constant  Value=-0.00016
  a_8 : Constant  Value=-8.88
  C_t : Outport
  wires:
  a_3/1 -> Product2/2
  beta/1 -> Product6/1, Product4/1, Product2/1, Product3/1
  a_1/1 -> Add/1
  Product1/1 -> Add/2
  Math Function5/1 -> Product5/3
  Gain3/1 -> Product6/2
  lambda/1 -> Math Function4/1, Math Function2/1, Subtract/1
  Math Function2/1 -> Product/1
  a_4/1 -> Gain1/1
  Product5/1 -> Add/4
  a_2/1 -> Product1/1
  Product3/1 -> Math Function1/1
  Product6/1 -> Math Function5/1
  Product4/1 -> Math Function3/1
  Math Function1/1 -> Product1/3
  Constant1/1 -> Math Function4/2
  Math Function4/1 -> Product5/2
  a_5/1 -> Product/2
  Add/1 -> Saturation/1
  Product2/1 -> Subtract/2
  Subtract/1 -> Product1/2
  Gain1/1 -> Product3/2
  a_7/1 -> Product5/1
  a_8/1 -> Gain3/1
  Gain2/1 -> Product4/2
  Math Function3/1 -> Product/3
  Product/1 -> Add/3
  a_6/1 -> Gain2/1
  Saturation/1 -> C_t/1

== system ControlSystems16/Yaw Control System/Aerodynamic Yaw Torque/block 2 ==
  Thrust_Coefficient : Inport
  wind_velocity : Inport  Port=2
  Wind Angle difference : Inport  Port=3
  0.5*A : Constant  Value=0.5*pi*35^2
  Gain : Gain  Gain=0.001
  Gain1 : Gain  Gain=0.5
  Math Function2 : Math  Operator=square  SaturateOnIntegerOverflow=on
  Product : Product
  Product1 : Product  Inputs=4
  Product2 : Product  Inputs=3
  Sign : Signum
  Subtract : Sum
  Yaw_Torque : Outport
  wires:
  0.5*A/1 -> Product2/1, Product1/1
  Thrust_Coefficient/1 -> Product2/2, Product1/2
  Math Function2/1 -> Product2/3, Product1/3
  wind_velocity/1 -> Math Function2/1
  Wind Angle difference/1 -> Product1/4, Sign/1
  Product2/1 -> Gain/1
  Product1/1 -> Subtract/2
  Subtract/1 -> Gain1/1
  Gain/1 -> Product/1
  Sign/1 -> Product/2
  Product/1 -> Subtract/1
  Gain1/1 -> Yaw_Torque/1

== system ControlSystems16/Drivetrain/Aerodynamic Block/Power Coefficient/Lamda i ==
  In1 : Inport
  In2 : Inport  Port=2
  Divide : Product  Inputs=*/
  Divide1 : Product  Inputs=*/
  Divide2 : Product  Inputs=*/
  Math Function : Math  Operator=magnitude^2  SaturateOnIntegerOverflow=on
  Product : Product
  Sum : Sum  Inputs=|+-
  Sum1 : Sum  Inputs=|+-
  Sum2 : Sum  Inputs=|++
  c8 : Gain  Gain=0.02
  c9 : Constant  Value=0.003
  one : Constant
  one1 : Constant
  Out1 : Outport
  wires:
  Divide/1 -> Out1/1
  In1/1 -> Sum1/1
  Product/1 -> Sum2/1
  Sum2/1 -> Divide2/2
  c8/1 -> Sum1/2
  Sum/1 -> Divide/2
  c9/1 -> Divide2/1
  Divide1/1 -> Sum/1
  Math Function/1 -> Product/1
  In2/1 -> Product/2, Math Function/1, c8/1
  one1/1 -> Sum2/2
  Divide2/1 -> Sum/2
  Sum1/1 -> Divide1/2
  one/1 -> Divide/1, Divide1/1

== system ControlSystems16/Drivetrain/Electricl Block/Thevenin Reactance/Mutual Reactance ==
  Gain3 : Gain  Gain=2*pi
  Mutual Inductance : Constant  Value=0.0007749
  Out1 : Outport
  wires:
  Gain3/1 -> Out1/1
  Mutual Inductance/1 -> Gain3/1

== system ControlSystems16/Drivetrain/Electricl Block/Thevenin Reactance/Stator Reactance ==
  Gain3 : Gain  Gain=2*pi
  Stator Inductance : Constant  Value=0.000195
  Out1 : Outport
  wires:
  Gain3/1 -> Out1/1
  Stator Inductance/1 -> Gain3/1

== system ControlSystems16/Drivetrain/Electricl Block/Thevenin Resistance/Mutual Reactance ==
  Gain3 : Gain  Gain=2*pi
  Mutual Inductance : Constant  Value=0.0007749
  Out1 : Outport
  wires:
  Gain3/1 -> Out1/1
  Mutual Inductance/1 -> Gain3/1

== system ControlSystems16/Drivetrain/Electricl Block/Thevenin Resistance/Stator Reactance ==
  Gain3 : Gain  Gain=2*pi
  Stator Inductance : Constant  Value=0.000195
  Out1 : Outport
  wires:
  Gain3/1 -> Out1/1
  Stator Inductance/1 -> Gain3/1

== system ControlSystems16/Drivetrain/Electricl Block/Thevenin Voltage/Mutual Reactance ==
  Gain3 : Gain  Gain=2*pi
  Mutual Inductance : Constant  Value=0.0007749
  Out1 : Outport
  wires:
  Gain3/1 -> Out1/1
  Mutual Inductance/1 -> Gain3/1

== system ControlSystems16/Drivetrain/Electricl Block/Thevenin Voltage/Stator Reactance ==
  Gain3 : Gain  Gain=2*pi
  Stator Inductance : Constant  Value=0.000195
  Out1 : Outport
  wires:
  Gain3/1 -> Out1/1
  Stator Inductance/1 -> Gain3/1
